simulink model "charges_pneus"  (R2024b)
settings: Solver=FixedStepAuto  StartTime=0.0  StopTime=10.0  FixedStep=Ts  MaxStep=0.001  RelTol=1e-3
values from neighbouring files (symbols this model uses):
  fr = 0.51    [main_data_vehicle.m]    (also in xopt_launch.mat)
  g = 9.81    [main_data_vehicle.m]    (also in xopt_launch.mat)
  h = 0.29    [main_data_vehicle.m]    (also in xopt_launch.mat)
  L = 1.55    [main_data_vehicle.m]    (also in xopt_launch.mat)
  m = 265    [main_data_vehicle.m]    (also in xopt_launch.mat)
settings Model: Creator=marti  LastModifiedBy=marti

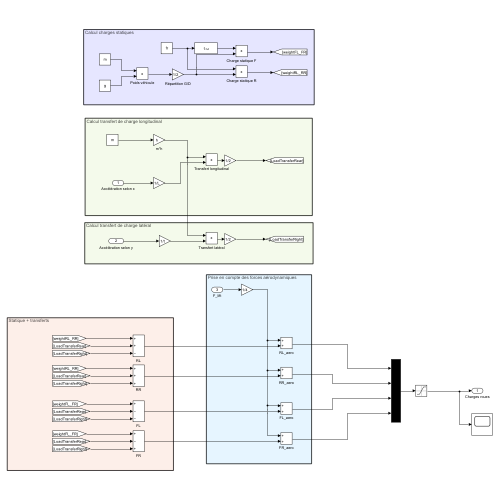
[thumbnail: Simulink's stored preview of the top-level diagram]
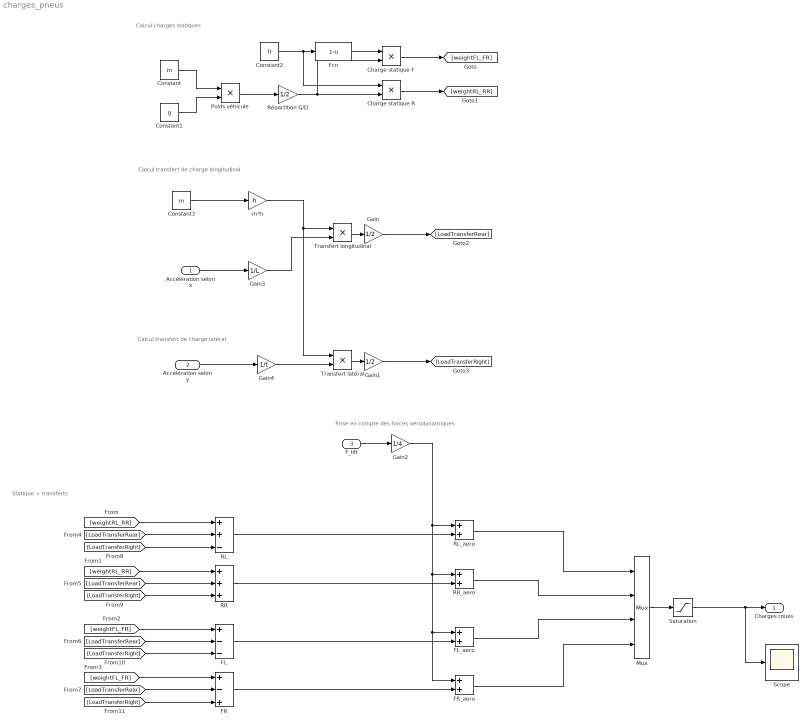
== system charges_pneus ==
  note: Prise en compte des forces aérodynamiques
  note: Statique + transferts
  note: Calcul transfert de charge latéral
  note: Calcul transfert de charge longitudinal
  note: Calcul charges statiques
  Accélération selon x : Inport
  Accélération selon y : Inport  Port=2
  F_lift : Inport  Port=3
  Charge statique F : Product
  Charge statique R : Product
  Constant : Constant  Value=m
  Constant1 : Constant  Value=g
  Constant2 : Constant  Value=fr
  Constant3 : Constant  Value=m
  FL : Sum  Inputs=+--
  FL_aero : Sum
  FR : Sum  Inputs=+-+
  FR_aero : Sum
  Fcn : Fcn  Expr=1-u
  Gain : Gain  Gain=1/2
  Gain1 : Gain  Gain=1/2
  Gain2 : Gain  Gain=1/4
  Gain3 : Gain  Gain=1/L
  Gain4 : Gain  Gain=1/t
  Mux : Mux
  Poids véhicule : Product
  RL : Sum  Inputs=++-
  RL_aero : Sum
  RR : Sum  Inputs=+++
  RR_aero : Sum
  Répartition G/D : Gain  Gain=1/2
  Saturation : Saturate  UpperLimit=m*g  LowerLimit=30
  Scope : Scope
  Transfert latéral : Product
  Transfert longitudinal : Product
  m*h : Gain  Gain=h
  Charges roues : Outport
  wires:
  Constant1/1 -> Poids véhicule/2
  Constant/1 -> Poids véhicule/1
  Poids véhicule/1 -> Répartition G/D/1
  Constant2/1 -> Charge statique R/1, Fcn/1
  Fcn/1 -> Charge statique F/1
  Répartition G/D/1 -> Charge statique F/2, Charge statique R/2
  Accélération selon x/1 -> Gain3/1
  Gain3/1 -> Transfert longitudinal/2
  m*h/1 -> Transfert longitudinal/1, Transfert latéral/1
  Accélération selon y/1 -> Gain4/1
  Gain4/1 -> Transfert latéral/2
  Transfert latéral/1 -> Gain1/1
  Transfert longitudinal/1 -> Gain/1
  RL/1 -> RL_aero/2
  RR/1 -> RR_aero/2
  FL/1 -> FL_aero/2
  FR/1 -> FR_aero/2
  F_lift/1 -> Gain2/1
  Gain2/1 -> FR_aero/1, FL_aero/1, RR_aero/1, RL_aero/1
  RL_aero/1 -> Mux/1
  RR_aero/1 -> Mux/2
  FL_aero/1 -> Mux/3
  FR_aero/1 -> Mux/4
  Mux/1 -> Saturation/1
  Charge statique F/1 -> [weightFL_FR]
  Charge statique R/1 -> [weightRL_RR]
  Constant3/1 -> m*h/1
  Gain/1 -> [LoadTransferRear]
  Gain1/1 -> [LoadTransferRight]
  [weightRL_RR] -> RL/1
  [weightRL_RR] -> RR/1
  [weightFL_FR] -> FL/1
  [weightFL_FR] -> FR/1
  [LoadTransferRear] -> RL/2
  [LoadTransferRear] -> RR/2
  [LoadTransferRear] -> FL/2
  [LoadTransferRear] -> FR/2
  [LoadTransferRight] -> RL/3
  [LoadTransferRight] -> RR/3
  [LoadTransferRight] -> FL/3
  [LoadTransferRight] -> FR/3
  Saturation/1 -> Scope/1, Charges roues/1
